simulink model "narx"  (R2019a)
settings: Solver=VariableStepAuto  StartTime=0.0  StopTime=10.0  RelTol=1e-3
libraries: neural x208
(part 3 of 4)

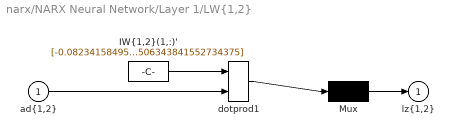
== system narx/NARX Neural Network/Layer 1/LW{1,2} ==
  "ad{1,2}" : Inport  PortDimensions=400  SampleTime=0.1
      mask Display: e = 0.06;c1 = [120 230 180]/255;c2 = ([120 230 180]+0)/(256+128);c3 = ([120 230 180]+128)/(256+128);patch([0 1 1 0],[0 0 1 1],c1);patch([0 1 1 1-e 1-e 0+e],[0 0 1 1-e 0+e 0+e],c2);patch([0 0 1 1-e 0+e 0+e],[0 1 1 1-e 1-e 0+e],c3);plot([0 1 1 0 0],[0 0 1 1 0]);
  "IW{1,2}(1,:)'" : Constant  Value=[-0.0823415849527278920216843971502385102212429046630859375;-0.01397174690725889144304883160430108546279370784759521484375;-0.029261430938860133466050683637149631977081298828125;-0.0256713793827941828828986814414747641421854496002197265625;-0.042725463936756795380045304000304895453155040740966796875;-0.01459398774548865442002298919987879344262182712554931640625;-0.0760191894158710190776417903180117718875408172607421875;0.07681585613294973635678530854420387186110019683837890625;-0.0778895894931407040129300867192796431481838226318359375;0.00648258834639818017075985068231602781452238559722900390625;0.004741280530683231360378204755079423193819820880889892578125;-0.0694701080912200341632711797501542605459690093994140625;-0.04483753132973684885076437467432697303593158721923828125;-0.019071088721181649050517847854280262254178524017333984375;-0.01206975959504176347525383761194461840204894542694091796875;0.047172920143841327866862656037483247928321361541748046875;0.060646391480755061642593517490240628831088542938232421875;0.07640034894099421991509046847568242810666561126708984375;-0.064110895658603006541653712702100165188312530517578125;-0.0523122425143255076473991493912762962281703948974609375;-0.06565779790903857049411129764848737977445125579833984375;-0.00701827770466369703361575460576204932294785976409912109375;-0.049857930088974544702296043396927416324615478515625;-0.03607921538989074250469712978883762843906879425048828125;-0.026428234513581512488133995475436677224934101104736328125;0.019454482471527978493242017066222615540027618408203125;0.02731547626172849130288255992127233184874057769775390625;0.08216117490734066441948613146450952626764774322509765625;-0.01224128796196832270892773664172636927105486392974853515625;0.057657207662517868940188492388188024051487445831298828125;-0.05201487812347938000101521538454107940196990966796875;-0.0177555924270427593902876850506800110451877117156982421875;0.0112586324361499123813956657613744027912616729736328125;0.0782838148993710569722992431707098148763179779052734375;-0.07667853437551576389896723640049458481371402740478515625;-0.07322890997823965075763652521345647983253002166748046875;0.07004799555301439994980938763546873815357685089111328125;0.0336485356403254665114133103998028673231601715087890625;0.06087105125894450019519155148373101837933063507080078125;0.04696065344609391678520893265158520080149173736572265625;0.0784892129181365694190475323921418748795986175537109375;-0.0192128198158475517465237913938835845328867435455322265625;-0.0126891611690110629739880465649548568762838840484619140625;-0.039902002214343125496842645816286676563322544097900390625;0.0002861175567481866817594327034868229020503349602222442626953125;-0.0825614706941331932821270811473368667066097259521484375;0.06502748801856329807780099372394033707678318023681640625;-0.028168430205081425310442710951974731869995594024658203125;-0.051243967658969789835676778011475107632577419281005859375;-0.036287046428123026498013814489240758121013641357421875;0.07713476015031439647628985767369158565998077392578125;0.0247201829615873412693272115348008810542523860931396484375;-0.036797041607220408454548277177309500984847545623779296875;-0.032019425735312280478783719672719598747789859771728515625;-0.00899356953221560305455906103588858968578279018402099609375;0.06720665539782820496750304073430015705525875091552734375;-0.0289447437565115255064807087137523922137916088104248046875;-0.0205898463785867645581273421839796355925500392913818359375;0.0474892330284455710387447879838873632252216339111328125;0.02744419530706228294025805780620430596172809600830078125;-0.08316606864860660863758567984405090101063251495361328125;-0.0693170834361665766376603414755663834512233734130859375;-0.041778713971127069692901301323217921890318393707275390625;-0.039764901446949794949770051744053489528596401214599609375;-0.06509088878715059423019084761108388192951679229736328125;-0.0001727264425261800331358463811426418033079244196414947509765625 ...(+20028 chars)]
      mask Display: e = 0.06;c1 = [120 150 230]/255;c2 = ([120 150 230]+0)/383;c3 = ([120 150 230]+128)/383;patch([0 1 1 0],[0 0 1 1],c1);patch([0 1 1 1-e 1-e 0+e],[0 0 1 1-e 0+e 0+e],c2);patch([0 0 1 1-e 0+e 0+e],[0 1 1 1-e 1-e 0+e],c3);plot([0 1 1 0 0],[0 0 1 1 0]);disp('weights');
  Mux : Mux  Inputs=1
      mask Display: e = 0.06;c1 = [120 150 230]/255;c2 = ([120 150 230]+0)/383;c3 = ([120 150 230]+128)/383;patch([0 1 1 0],[0 0 1 1],c1);patch([0 1 1 1-e 1-e 0+e],[0 0 1 1-e 0+e 0+e],c2);patch([0 0 1 1-e 0+e 0+e],[0 1 1 1-e 1-e 0+e],c3);plot([0 1 1 0 0],[0 0 1 1 0]);disp('Mux');
  dotprod1 : neural/Weight Functions/dotprod
      settings: SourceProductName=MATLAB Runtime - Deep Learning Toolbox  SourceProductBaseCode=Missing
  "lz{1,2}" : Outport
      mask Display: e = 0.06;c1 = [120 230 180]/255;c2 = ([120 230 180]+0)/(256+128);c3 = ([120 230 180]+128)/(256+128);patch([0 1 1 0],[0 0 1 1],c1);patch([0 1 1 1-e 1-e 0+e],[0 0 1 1-e 0+e 0+e],c2);patch([0 0 1 1-e 0+e 0+e],[0 1 1 1-e 1-e 0+e],c3);plot([0 1 1 0 0],[0 0 1 1 0]);
  wires:
  "IW{1,2}(1,:)'"/1 -> dotprod1/1
  "ad{1,2}"/1 -> dotprod1/2
  dotprod1/1 -> Mux/1
  Mux/1 -> "lz{1,2}"/1

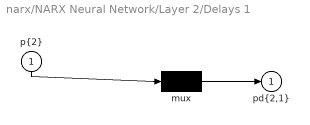
== system narx/NARX Neural Network/Layer 2/Delays 1 ==
  "p{2}" : Inport  PortDimensions=1  SampleTime=0.1
      mask Display: e = 0.06;c1 = [120 230 180]/255;c2 = ([120 230 180]+0)/(256+128);c3 = ([120 230 180]+128)/(256+128);patch([0 1 1 0],[0 0 1 1],c1);patch([0 1 1 1-e 1-e 0+e],[0 0 1 1-e 0+e 0+e],c2);patch([0 0 1 1-e 0+e 0+e],[0 1 1 1-e 1-e 0+e],c3);plot([0 1 1 0 0],[0 0 1 1 0]);
  mux : Mux  Inputs=1
      mask Display: e = 0.06;c1 = [120 150 230]/255;c2 = ([120 150 230]+0)/383;c3 = ([120 150 230]+128)/383;patch([0 1 1 0],[0 0 1 1],c1);patch([0 1 1 1-e 1-e 0+e],[0 0 1 1-e 0+e 0+e],c2);patch([0 0 1 1-e 0+e 0+e],[0 1 1 1-e 1-e 0+e],c3);plot([0 1 1 0 0],[0 0 1 1 0]);disp('Mux')
  "pd{2,1}" : Outport
      mask Display: e = 0.06;c1 = [120 230 180]/255;c2 = ([120 230 180]+0)/(256+128);c3 = ([120 230 180]+128)/(256+128);patch([0 1 1 0],[0 0 1 1],c1);patch([0 1 1 1-e 1-e 0+e],[0 0 1 1-e 0+e 0+e],c2);patch([0 0 1 1-e 0+e 0+e],[0 1 1 1-e 1-e 0+e],c3);plot([0 1 1 0 0],[0 0 1 1 0]);
  wires:
  "p{2}"/1 -> mux/1
  mux/1 -> "pd{2,1}"/1
